simulink model "Reaction_model_simulink_1_2"  (R2025b)
settings: Solver=VariableStepAuto  StartTime=0.0  StopTime=200  RelTol=1e-3
undefined symbols (not defined in the file or in its folder): Den, Jr, Num, Tc_max, wr_max
libraries: SignalEditorBlockLib x1
settings Model: Creator=flori  LastModifiedBy=flori

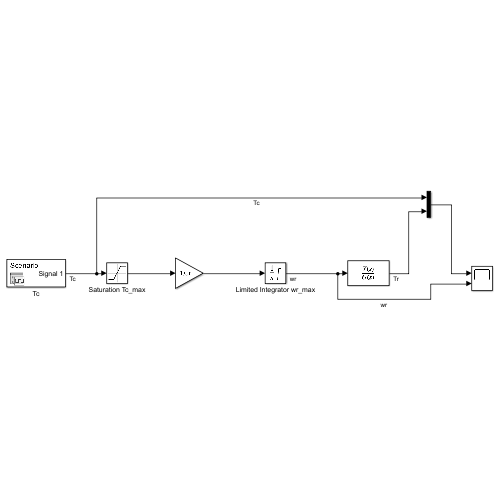
[thumbnail: Simulink's stored preview of the top-level diagram]
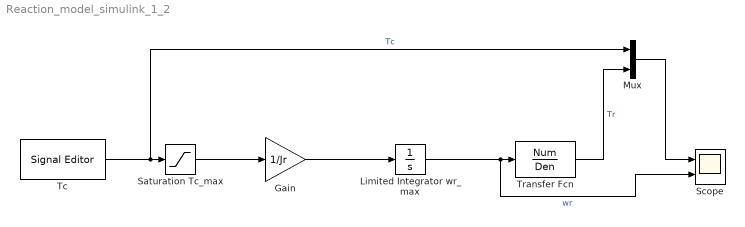
== system Reaction_model_simulink_1_2 ==
  Gain : Gain  Gain=1/Jr
  Limited Integrator wr_max : Integrator  LimitOutput=on  UpperSaturationLimit=wr_max  LowerSaturationLimit=-wr_max
  Mux : Mux  Inputs=2
  Saturation Tc_max : Saturate  UpperLimit=Tc_max  LowerLimit=-Tc_max
  Scope : Scope  NumInputPorts=2
      settings: ActiveDisplayYMinimum=-0.0037918684967391644  ActiveDisplayYMaximum=0.0041268164706524807  DataLoggingVariableName=reaction_wheel_scope
  Tc : SignalEditorBlockLib/Signal Editor  FileName=square signal.mat  ActiveScenario=Scenario  ActiveSignal=Signal 1  IsBus=off  OutputBusObjectStr=Bus: BusObject  SampleTime=0  ZeroCross=off  OutputAfterFinalValue=Setting to zero  Unit=inherit  PreserveSignalName=on  ApplySigPropsToAllScenarios=off  ApplySigPropsToAllSignals=off  SignalPropertySource=Signal data in MAT file
  Transfer Fcn : TransferFcn  Numerator=Num  Denominator=Den
  wires:
  Saturation Tc_max/1 -> Gain/1
  Gain/1 -> Limited Integrator wr_max/1
  Limited Integrator wr_max/1 -> Scope/2, Transfer Fcn/1  "wr"
  Tc/1 -> Mux/1, Saturation Tc_max/1  "Tc"
  Transfer Fcn/1 -> Mux/2  "Tr"
  Mux/1 -> Scope/1
